simulink model "lyskawaLab7_si_nonlinear"  (R2023b)
settings: Solver=VariableStepAuto  StartTime=startTime  StopTime=stopTime  MaxStep=maxStepSize  RelTol=1e-3
values from neighbouring files (symbols this model uses):
  A1 = 2    [lyskawaLab7.m]
  A2 = 2    [lyskawaLab7.m]
  Aw1 = 0.1 * 2    (= 0.2)    [lyskawaLab7.m]
  Aw2 = 0.1 * 2    (= 0.2)    [lyskawaLab7.m]
  dfwe1 = 0    [lyskawaLab7.m]
  dfwe2 = 0.1*fwe2max    [lyskawaLab7.m]
  fwe1_0 = 0.2 * fwe1max    [lyskawaLab7.m]
  fwe2_0 = arrayfwe2_0(i)    [lyskawaLab7.m]
  g = 9.81    [lyskawaLab7.m]
  h1_0 = (fwe1_0^2)/(Aw1^2 *2*g) + h2_0    [lyskawaLab7.m]
  h2_0 = (fwe1_0+fwe2_0)^2/(Aw2^2 *2*g)    [lyskawaLab7.m]
  t0 = 5    [lyskawaLab7.m]
settings Model: Creator=aleklyskawa  LastModifiedBy=aleklyskawa

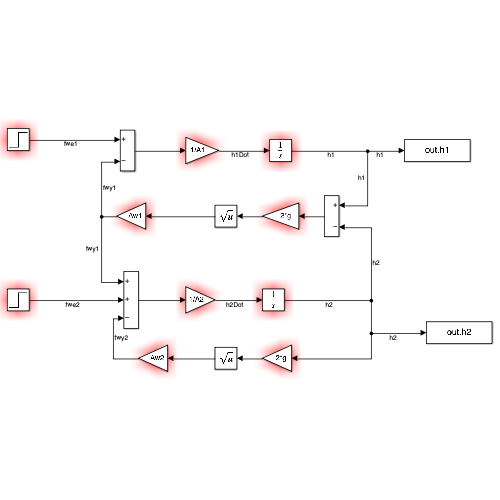
[thumbnail: Simulink's stored preview of the top-level diagram]
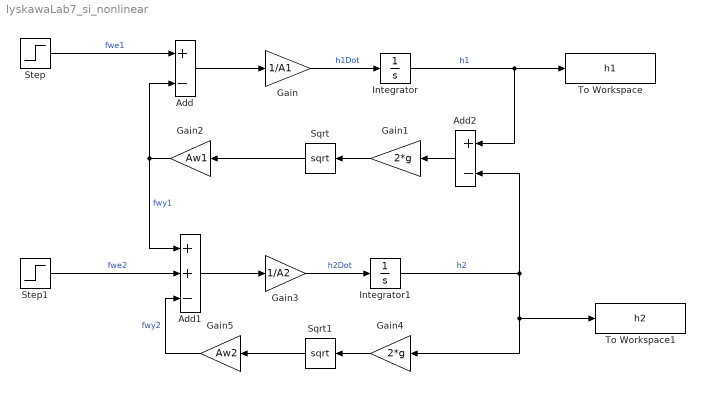
== system lyskawaLab7_si_nonlinear ==
  Add : Sum  Inputs=+-
  Add1 : Sum  Inputs=++-
  Add2 : Sum  Inputs=+-
  Gain : Gain  Gain=1/A1
  Gain1 : Gain  Gain=2*g
  Gain2 : Gain  Gain=Aw1
  Gain3 : Gain  Gain=1/A2
  Gain4 : Gain  Gain=2*g
  Gain5 : Gain  Gain=Aw2
  Integrator : Integrator  InitialCondition=h1_0
  Integrator1 : Integrator  InitialCondition=h2_0
  Sqrt : Sqrt
  Sqrt1 : Sqrt
  Step : Step  Time=t0  Before=fwe1_0  After=fwe1_0+dfwe1  SampleTime=0
  Step1 : Step  Time=t0  Before=fwe2_0  After=fwe2_0+dfwe2  SampleTime=0
  To Workspace : ToWorkspace  VariableName=h1  SampleTime=-1
  To Workspace1 : ToWorkspace  VariableName=h2  SampleTime=-1
  wires:
  Gain1/1 -> Sqrt/1
  Integrator/1 -> Add2/1, To Workspace/1  "h1"
  Gain4/1 -> Sqrt1/1
  Gain/1 -> Integrator/1  "h1Dot"
  Gain5/1 -> Add1/3  "fwy2"
  Step/1 -> Add/1  "fwe1"
  Gain3/1 -> Integrator1/1  "h2Dot"
  Add/1 -> Gain/1
  Integrator1/1 -> To Workspace1/1, Gain4/1, Add2/2  "h2"
  Add2/1 -> Gain1/1
  Step1/1 -> Add1/2  "fwe2"
  Gain2/1 -> Add1/1, Add/2  "fwy1"
  Add1/1 -> Gain3/1
  Sqrt/1 -> Gain2/1
  Sqrt1/1 -> Gain5/1
